simulink model "inv_pend_damp"  (R2019a)
settings: Solver=VariableStepAuto  StartTime=0.0  StopTime=100  MaxStep=0.01  RelTol=1e-3  EnableMultiTasking=on
InitFcn:
  | init
undefined symbols (not defined in the file): b, g, J, l, m
libraries: simulink_extras x1
settings Model: Creator=roslovetspv  LastModifiedBy=Pavel Roslovets
settings OptimizationCC: LifeSpan=inf
settings DebuggingCC: SFUnexpectedBacktrackingDiag=warning  SFNoUnconditionalDefaultTransitionDiag=warning  SFExecutionAtInitializationDiag=none  ArithmeticOperatorsInVariantConditions=warning
settings SFSimCC: SimUseLocalCustomCode=off
settings RTWCC: RTWUseLocalCustomCode=off
settings CodeAppCC: StateflowObjectComments=on
settings GRTTargetCC: TargetLangStandard=C89/C90 (ANSI)  GeneratePreprocessorConditionals=Disable all
settings ConfigComp: CovMetricSettings=dw  CovHtmlReporting=on  CovSaveCumulativeToWorkspaceVar=on  CovSaveSingleToWorkspaceVar=on  CovExternalEMLEnable=off

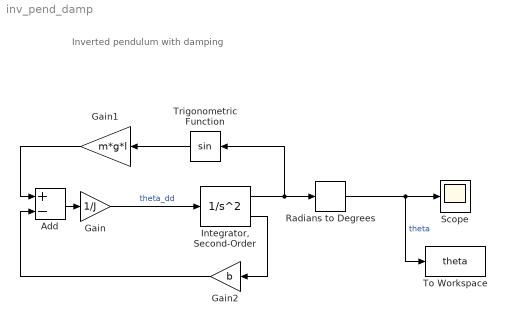
== system inv_pend_damp ==
  note: Inverted pendulum with damping
  Add : Sum  Inputs=+-
  Gain : Gain  Gain=1/J
  Gain1 : Gain  Gain=m*g*l
  Gain2 : Gain  Gain=b
  "Integrator, Second-Order" : SecondOrderIntegrator  ICX=0.01
  Radians to Degrees : simulink_extras/Transformations/Radians to Degrees
  Scope : Scope
  To Workspace : ToWorkspace  VariableName=theta  SampleTime=-1
  Trigonometric Function : Trigonometry
  wires:
  Radians to Degrees/1 -> To Workspace/1, Scope/1  "theta"
  "Integrator, Second-Order"/1 -> Trigonometric Function/1, Radians to Degrees/1
  Gain/1 -> "Integrator, Second-Order"/1  "theta_dd"
  Trigonometric Function/1 -> Gain1/1
  Gain1/1 -> Add/1
  Add/1 -> Gain/1
  "Integrator, Second-Order"/2 -> Gain2/1
  Gain2/1 -> Add/2
